simulink library "dyn"  (Simulink 8.2)
settings: Solver=ode45  StartTime=0.0  StopTime=10.0  RelTol=1e-3
undefined symbols (not defined in the file or in its folder): KVSE_AccelWeightOffset_rat, KVSE_AccelWeightSlope_rat, KVSE_StartModeInDelaySpd_kph, KVSE_StartModeInWheelSpd_kph, KVSE_StartModeOutWheelSpd_kph, KVSE_TurnModeInYawRate_degps, KVSE_TurnModeOutYawRate_degps, KVSE_WheelSpdAdjust_rat, KVSE_WheelWeightOffset_rat, KVSE_WheelWeightSlope_rat
libraries: simulink x6
(part 2 of 2)

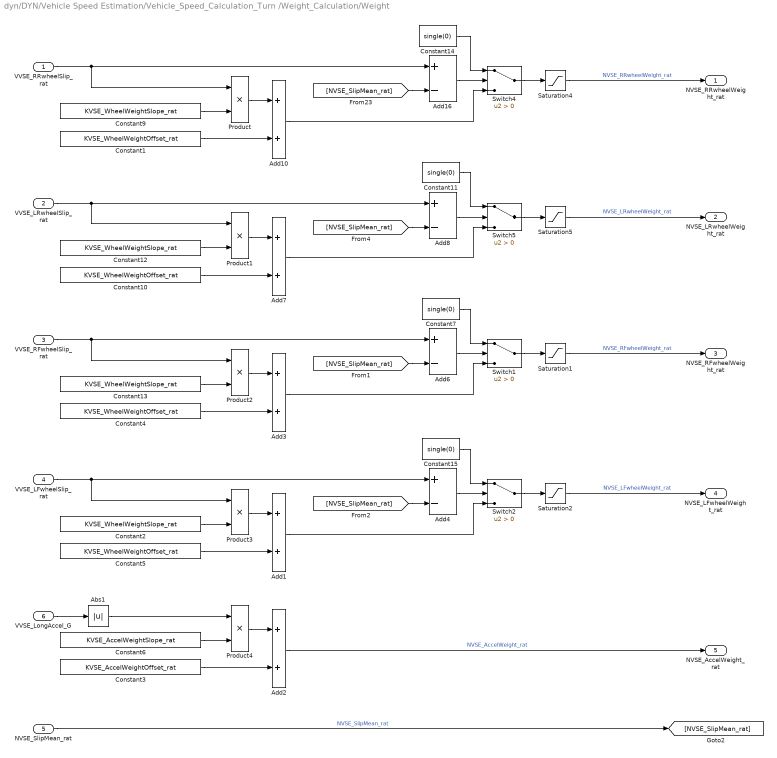
== system dyn/DYN/Vehicle Speed Estimation/Vehicle_Speed_Calculation_Turn /Weight_Calculation/Weight ==
  VVSE_RRwheelSlip_rat : Inport
  VVSE_LRwheelSlip_rat : Inport  Port=2
  VVSE_RFwheelSlip_rat : Inport  Port=3
  VVSE_LFwheelSlip_rat : Inport  Port=4
  NVSE_SlipMean_rat : Inport  Port=5
  VVSE_LongAccel_G : Inport  Port=6
  Abs1 : Abs
  Add{1..3,7,10} (5 alike) : Sum
  Add{4,6,8,16} (4 alike) : Sum  Inputs=+-
  Constant{1,4..5,10} (4 alike) : Constant  Value=KVSE_WheelWeightOffset_rat
  Constant{7,11,14..15} (4 alike) : Constant  Value=single(0)
  Constant{2,9,12..13} (4 alike) : Constant  Value=KVSE_WheelWeightSlope_rat
  Constant3 : Constant  Value=KVSE_AccelWeightOffset_rat
  Constant6 : Constant  Value=KVSE_AccelWeightSlope_rat
  Product{,1..4} (5 alike) : Product
  Saturation{1..2,4..5} (4 alike) : Saturate  UpperLimit=Inf  LowerLimit=0
  Switch{1..2,4..5} (4 alike) : Switch  Criteria=u2 > Threshold
  NVSE_RRwheelWeight_rat : Outport
  NVSE_LRwheelWeight_rat : Outport  Port=2
  NVSE_RFwheelWeight_rat : Outport  Port=3
  NVSE_LFwheelWeight_rat : Outport  Port=4
  NVSE_AccelWeight_rat : Outport  Port=5
  wires:
  Constant6/1 -> Product4/2
  Product4/1 -> Add2/1
  Constant2/1 -> Product3/2
  Switch2/1 -> Saturation2/1
  Saturation2/1 -> NVSE_LFwheelWeight_rat/1  "NVSE_LFwheelWeight_rat"
  VVSE_LFwheelSlip_rat/1 -> Add4/1, Product3/1
  Constant5/1 -> Add1/2
  Product3/1 -> Add1/1
  Constant15/1 -> Switch2/1
  Add1/1 -> Switch2/3
  Add4/1 -> Switch2/2
  [NVSE_SlipMean_rat] -> Add4/2
  Constant13/1 -> Product2/2
  Switch1/1 -> Saturation1/1
  Saturation1/1 -> NVSE_RFwheelWeight_rat/1  "NVSE_RFwheelWeight_rat"
  VVSE_RFwheelSlip_rat/1 -> Add6/1, Product2/1
  Constant4/1 -> Add3/2
  Product2/1 -> Add3/1
  Constant7/1 -> Switch1/1
  Add3/1 -> Switch1/3
  Add6/1 -> Switch1/2
  [NVSE_SlipMean_rat] -> Add6/2
  Constant12/1 -> Product1/2
  Switch5/1 -> Saturation5/1
  Saturation5/1 -> NVSE_LRwheelWeight_rat/1  "NVSE_LRwheelWeight_rat"
  VVSE_LRwheelSlip_rat/1 -> Add8/1, Product1/1
  Constant10/1 -> Add7/2
  Product1/1 -> Add7/1
  Constant11/1 -> Switch5/1
  Add7/1 -> Switch5/3
  Add8/1 -> Switch5/2
  [NVSE_SlipMean_rat] -> Add8/2
  Constant9/1 -> Product/2
  Constant3/1 -> Add2/2
  Switch4/1 -> Saturation4/1
  Saturation4/1 -> NVSE_RRwheelWeight_rat/1  "NVSE_RRwheelWeight_rat"
  VVSE_RRwheelSlip_rat/1 -> Add16/1, Product/1
  Constant1/1 -> Add10/2
  Product/1 -> Add10/1
  Add2/1 -> NVSE_AccelWeight_rat/1  "NVSE_AccelWeight_rat"
  Constant14/1 -> Switch4/1
  Add10/1 -> Switch4/3
  Add16/1 -> Switch4/2
  Abs1/1 -> Product4/1
  NVSE_SlipMean_rat/1 -> [NVSE_SlipMean_rat]  "NVSE_SlipMean_rat"
  [NVSE_SlipMean_rat] -> Add16/2
  VVSE_LongAccel_G/1 -> Abs1/1

== stateflow chart DYN/Vehicle Speed Estimation/Chart ==
  state start
    state land
      en:
      VVSE_SpdEstState_enum=uint8(1);
    state slope
      en:
      VVSE_SpdEstState_enum=uint8(1);
    (default) -> land
    land -> (junction 9) : [VVSE_LongAccel_G~=0]
    (junction 9) -> slope
    (junction 10) -> land
    slope -> (junction 10) : [VVSE_LongAccel_G==0]
  state nomal
    state straight
      en:
      VVSE_SpdEstState_enum=uint8(2);
    state turn
      en:
      VVSE_SpdEstState_enum=uint8(3);
    (default) -> straight
    straight -> (junction 16) : [abs(VVSE_YawRate_degps)>=KVSE_TurnModeInYawRate_degps]
    (junction 16) -> turn
    (junction 17) -> straight
    turn -> (junction 17) : [abs(VVSE_YawRate_degps)<KVSE_TurnModeOutYawRate_degps]
  (default) -> start
  nomal -> start : [VVSE_RRwheelSpd_kph<KVSE_StartModeInWheelSpd_kph...
      | & VVSE_LRwheelSpd_kph<KVSE_StartModeInWheelSpd_kph...
      | & VVSE_RFwheelSpd_kph<KVSE_StartModeInWheelSpd_kph...
      | & VVSE_LFwheelSpd_kph<KVSE_StartModeInWheelSpd_kph...
      | & VVSE_DelaySpd_kph<KVSE_StartModeInDelaySpd_kph]
  start -> nomal : [VVSE_RRwheelSpd_kph>KVSE_StartModeOutWheelSpd_kph...
      | ||VVSE_LRwheelSpd_kph>KVSE_StartModeOutWheelSpd_kph...
      | ||VVSE_RFwheelSpd_kph>KVSE_StartModeOutWheelSpd_kph...
      | ||VVSE_LFwheelSpd_kph>KVSE_StartModeOutWheelSpd_kph]
  data: VVSE_RRwheelSpd_kph input double; VVSE_LRwheelSpd_kph input double; VVSE_RFwheelSpd_kph input double; VVSE_LFwheelSpd_kph input double; VVSE_LongAccel_G input double; VVSE_DelaySpd_kph input double; VVSE_YawRate_degps input double; VVSE_SpdEstState_enum output double; KVSE_StartModeInWheelSpd_kph input double; KVSE_StartModeInDelaySpd_kph input double; KVSE_StartModeOutWheelSpd_kph input double; KVSE_TurnModeInYawRate_degps input double; KVSE_TurnModeOutYawRate_degps input double
